simulink model "NSMC_HOSMO_NDO"  (R2021b)
settings: Solver=ode5  StartTime=0.0  StopTime=20  FixedStep=10^(-4)  MaxStep=10-4  RelTol=1e-3
settings Model: Creator=wkw  LastModifiedBy=wkw

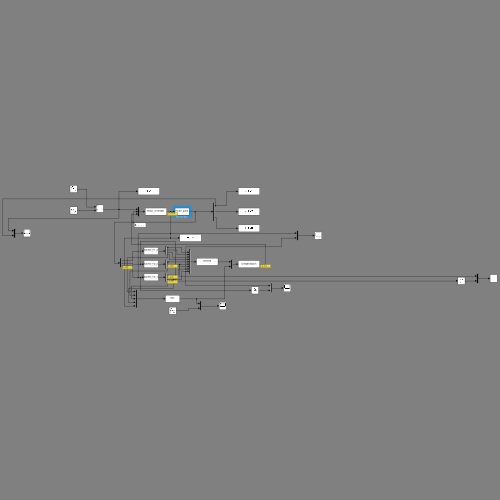
[thumbnail: Simulink's stored preview of the top-level diagram]
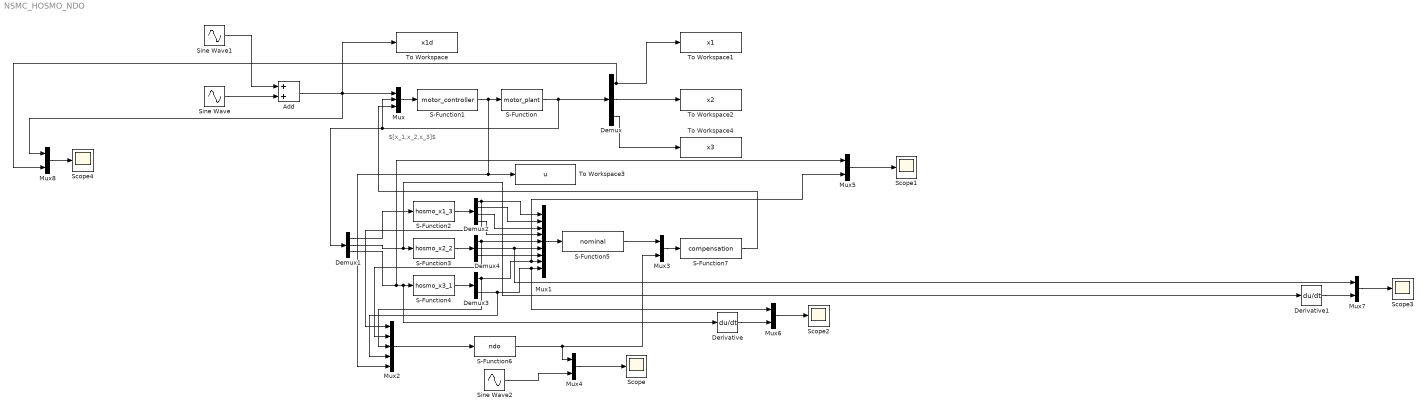
== system NSMC_HOSMO_NDO ==
  note: $[x_1,x_2,x_3]$
  Add : Sum
  Demux : Demux  Outputs=3
  Demux1 : Demux  Outputs=3
  Demux2 : Demux
  Demux3 : Demux  Outputs=2
  Demux4 : Demux  Outputs=3
  Derivative : Derivative
  Derivative1 : Derivative
  Mux : Mux  Inputs=3
  Mux1 : Mux  Inputs=9
  Mux2 : Mux  Inputs=5
  Mux{3..8} (6 alike) : Mux  Inputs=2
  S-Function : S-Function  FunctionName=motor_plant  SFunctionDeploymentMode=off  EnableBusSupport=off
  S-Function1 : S-Function  FunctionName=motor_controller  SFunctionDeploymentMode=off  EnableBusSupport=off
  S-Function2 : S-Function  FunctionName=hosmo_x1_3  SFunctionDeploymentMode=off  EnableBusSupport=off
  S-Function3 : S-Function  FunctionName=hosmo_x2_2  SFunctionDeploymentMode=off  EnableBusSupport=off
  S-Function4 : S-Function  FunctionName=hosmo_x3_1  SFunctionDeploymentMode=off  EnableBusSupport=off
  S-Function5 : S-Function  FunctionName=nominal  SFunctionDeploymentMode=off  EnableBusSupport=off
  S-Function6 : S-Function  FunctionName=ndo  SFunctionDeploymentMode=off  EnableBusSupport=off
  S-Function7 : S-Function  FunctionName=compensation  SFunctionDeploymentMode=off  EnableBusSupport=off
  Scope{,1..4} (5 alike) : Scope
  Sine Wave : Sin  Amplitude=0.5  SampleTime=0
  Sine Wave1 : Sin  Amplitude=0.5  Frequency=0.5  SampleTime=0
  Sine Wave2 : Sin  Amplitude=0.8  SampleTime=0
  To Workspace : ToWorkspace  VariableName=x1d  SaveFormat=Timeseries  SampleTime=-1
  To Workspace1 : ToWorkspace  VariableName=x1  SaveFormat=Timeseries  SampleTime=-1
  To Workspace2 : ToWorkspace  VariableName=x2  SaveFormat=Timeseries  SampleTime=-1
  To Workspace3 : ToWorkspace  VariableName=u  SaveFormat=Timeseries  SampleTime=-1
  To Workspace4 : ToWorkspace  VariableName=x3  SaveFormat=Timeseries  SampleTime=-1
  wires:
  Mux/1 -> S-Function1/1
  S-Function/1 -> Demux/1, Demux1/1, Mux/2
  S-Function1/1 -> Mux2/5, To Workspace3/1, S-Function/1
  Demux/1 -> Mux8/2, To Workspace1/1
  Demux/2 -> To Workspace2/1
  Demux/3 -> To Workspace4/1
  Add/1 -> Mux8/1, To Workspace/1, Mux/1
  Sine Wave/1 -> Add/2
  Sine Wave1/1 -> Add/1
  Demux1/1 -> S-Function2/1
  Demux1/2 -> Derivative1/1, S-Function3/1
  Demux1/3 -> Mux5/1, Derivative/1, S-Function4/1
  Mux1/1 -> S-Function5/1
  S-Function2/1 -> Demux2/1
  S-Function3/1 -> Demux4/1
  S-Function4/1 -> Demux3/1
  Demux2/1 -> Mux2/1, Mux1/1
  Demux2/2 -> Mux1/2
  Demux2/3 -> Mux1/3
  Demux2/4 -> Mux1/4
  Demux4/1 -> Mux2/2, Mux1/5
  Demux4/3 -> Mux1/7
  Demux3/1 -> Mux2/3, Mux5/2, Mux1/8
  Demux3/2 -> Mux2/4, Mux6/1, Mux1/9
  Mux2/1 -> S-Function6/1
  Mux3/1 -> S-Function7/1
  S-Function5/1 -> Mux3/1
  S-Function6/1 -> Mux4/1, Mux3/2
  S-Function7/1 -> Mux/3
  Mux4/1 -> Scope/1
  Sine Wave2/1 -> Mux4/2
  Mux5/1 -> Scope1/1
  Mux6/1 -> Scope2/1
  Derivative/1 -> Mux6/2
  Derivative1/1 -> Mux7/2
  Mux7/1 -> Scope3/1
  Demux4/2 -> Mux1/6, Mux7/1
  Mux8/1 -> Scope4/1
